simulink model "mcb_pmsm_foc_inductive_position_dsPIC33CK256MP508"  (R2023a)
settings: Solver=FixedStepDiscrete  StartTime=0.0  StopTime=10.0  FixedStep=50e-6  RelTol=1e-3  EnableMultiTasking=on
PreLoadFcn:
  | mcb_pmsm_foc_inductive_position_dsPIC33_data
PostLoadFcn:
  | mcb_pmsm_foc_inductive_position_dsPIC33_data
InitFcn:
  | mcb_pmsm_foc_inductive_position_dsPIC33_data
values from neighbouring files (symbols this model uses):
  PI_params = mcb.internal.SetControllerParameters(pmsm,inverter,PU_System,T_pwm,Ts,Ts_speed)    [dsPIC33CK256MP508_IPS_LVMC_sh.m]    (also in mcb_pmsm_foc_inductive_position_dsPIC33_data.m)
  PU_System = mcb_SetPUSystem(pmsm,inverter)    [dsPIC33CK256MP508_IPS_LVMC_sh.m]    (also in mcb_pmsm_foc_inductive_position_dsPIC33_data.m)
  PWM_frequency = 20e3    (= 20000)    [dsPIC33CK256MP508_IPS_LVMC_sh.m]    (also in mcb_pmsm_foc_inductive_position_dsPIC33_data.m)
  Ts = T_pwm    (= 5e-05)    [dsPIC33CK256MP508_IPS_LVMC_sh.m]    (also in mcb_pmsm_foc_inductive_position_dsPIC33_data.m)
  Ts_speed = 30*Ts    (= 0.0015)    [dsPIC33CK256MP508_IPS_LVMC_sh.m]    (also in mcb_pmsm_foc_inductive_position_dsPIC33_data.m)
undefined symbols (not defined in the file or in its folder): A0, A4, AN0, AN1, B0, B2, C12, C13, C14, C7, D11, D12, D13, D14, D5, D6, D7, DiscIntNeverNeededParam, inverter, Max, MaxPer, ms, NumBits1, NumBits2, P20, P32, P55, P60, P61, P62, P69, P70, P71, P75, P76, P77, P78, Pin, pmsm, PWM1max, Resol, s, us
libraries: simulink x29, MCHP_Blockset x22, mcbcontrolslib x7, slpidlib x3
(part 1 of 4)
settings Model: ExtModeBatchMode=on  ExtModeEnableFloating=off  ExtModeTrigDuration=32  Creator=I50990  LastModifiedBy=I50990
settings SolverCC: AutoInsertRateTranBlk=on
settings OptimizationCC: DefaultParameterBehavior=Inlined  DefaultUnderspecifiedDataType=single  InlineInvariantSignals=on  ReuseModelBlockBuffer=off  EnhancedBackFolding=on  StrengthReduction=on  BooleansAsBitfields=on  PassReuseOutputArgsAs=Individual arguments  ZeroExternalMemoryAtStartup=off  ZeroInternalMemoryAtStartup=off  OptimizeBlockOrder=speed  DifferentSizesBufferReuse=on  EfficientTunableParamExpr=on
settings DebuggingCC: MultiTaskDSMMsg=none  MultiTaskCondExecSysMsg=none  MultiTaskRateTransMsg=warning  ParameterOverflowMsg=none  ParameterPrecisionLossMsg=none  ParameterTunabilityLossMsg=error
settings HardwareCC: ProdBitPerInt=16  ProdBitPerPointer=16  ProdBitPerSizeT=16  ProdBitPerPtrDiffT=32  ProdLargestAtomicInteger=Integer  ProdLargestAtomicFloat=None  ProdWordSize=16  ProdLongLongMode=on  ProdHWDeviceType=Generic->Custom
settings ModelReferenceCC: ModelReferenceNumInstancesAllowed=Single
settings SFSimCC: MATLABDynamicMemAlloc=off
settings RTWCC: Description=Microchip Embedded Target PIC24 dsPIC30 dsPIC33 (real-time)  SystemTargetFile=MCHP_dsPIC_stf.tlc  TLCOptions="-aExtModeXCPClassicInterface=0  -aCreateExtModeTypes=1 -aExtModeXCPSimulationTimeInTicks=1"  TemplateMakefile=MCHP_dsPIC.tmf
settings CodeAppCC: ForceParamTrailComments=on  IgnoreCustomStorageClasses=off  MaxIdLength=255  OperatorAnnotations=on  SimulinkDataObjDesc=on  SFDataObjDesc=on  InsertBlockDesc=on
settings STFCustomTargetCC: TargetLibSuffix=_lib.a  TargetLangStandard=C89/C90 (ANSI)  CodeReplacementLibrary=Microchip Code Replacement Library for dsPIC  MultiwordLength=256  ConcurrentExecutionCompliant=off  CombineOutputUpdateFcns=on  CombineSignalStateStructs=on  SuppressErrorStatus=on  ERTCustomFileBanners=on  SupportNonFinite=off  SupportContinuousTime=off  RemoveResetFunc=on  MATLABClassNameForMDSCustomization=Simulink.SoftwareTarget.ERTCustomization  GRTInterface=off  UseToolchainInfoCompliant=off  SystemTargetFile=MCHP_dsPIC_stf.tlc
settings ERTTargetCC: TargetLibSuffix=_lib.a  CodeReplacementLibrary=Microchip Code Replacement Library for dsPIC  ParMdlRefBuildCompliant=off  CompOptLevelCompliant=off  ConcurrentExecutionCompliant=off  CombineSignalStateStructs=on  SuppressErrorStatus=on  SupportNonFinite=off  SupportNonInlinedSFcns=on  ModelStepFunctionPrototypeControlCompliant=off  CPPClassGenCompliant=off  UseToolchainInfoCompliant=off  ExtModeTransport=1  ExtModeStaticAlloc=on  ExtModeAutomaticAllocSize=off  ExtModeStaticAllocSize=2048  ExtModeMexFile=ext_xcp  ExtModeMexArgs=1 0 4000000 './MCHP_LVMC_template.X/MCHP_LVMC_template.elf'  ExtModeIntrfLevel=Level2 - Open  InlinedParameterPlacement=NonHierarchical  ERTSrcFileBannerTemplate=MCHP_dsPIC_code_template.cgt  ERTHdrFileBannerTemplate=MCHP_dsPIC_code_template.cgt  ERTDataSrcFileTemplate=MCHP_dsPIC_code_template.cgt  ERTDataHdrFileTemplate=MCHP_dsPIC_code_template.cgt  ERTCustomFileTemplate=MCHP_main.tlc  MaxLineWidth=110

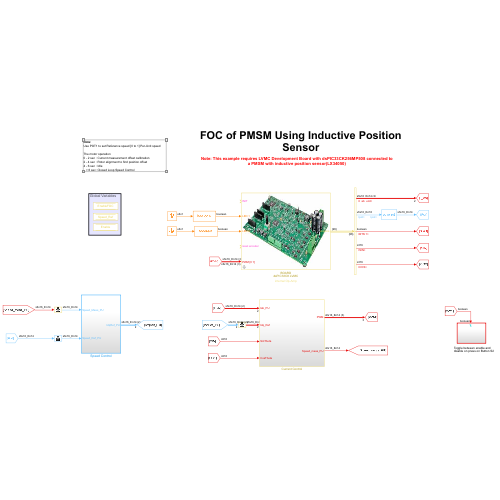
[thumbnail: Simulink's stored preview of the top-level diagram]
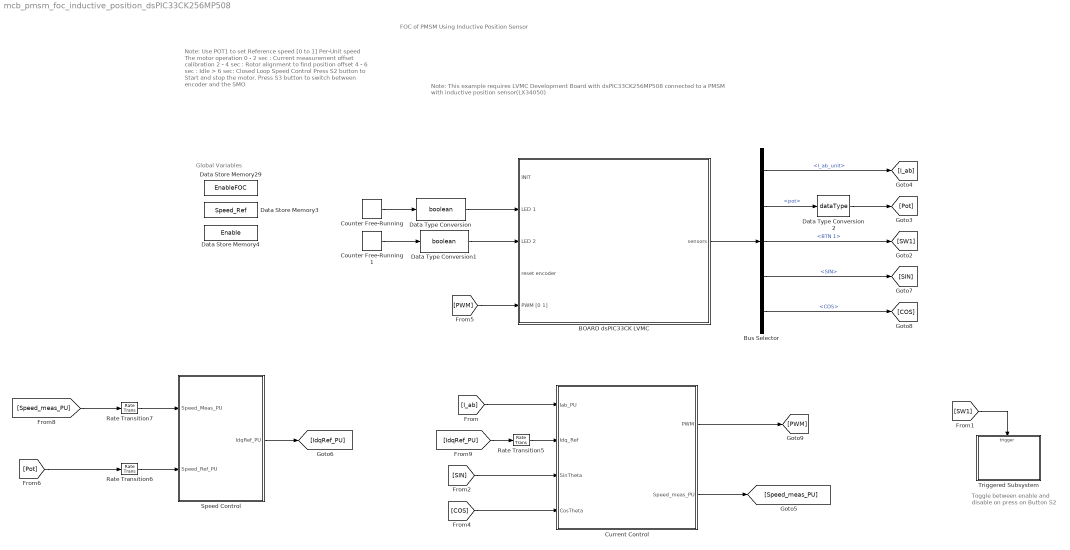
== system mcb_pmsm_foc_inductive_position_dsPIC33CK256MP508 ==
  note: Note:
      | Use POT1 to set Reference speed [0 to 1] Per-Unit speed
      |
      | The motor operation
      | 0 - 2 sec : Current measurement offset calibration
      | 2 - 4 sec : Rotor alignment to find position offset
      | 4 - 6 sec : Idle
      | > 6 sec: Closed Loop Speed Control
      |
      | Press S2 button to Start and stop the motor.
      | Press S3 button to switch between encoder and the SMO
  note: FOC of PMSM Using Inductive Position Sensor
  note: Note: This example requires LVMC Development Board with dsPIC33CK256MP508 connected to a PMSM with inductive position sensor(LX34050)
  note: Toggle between enable and disable on press on Button S2
  note: Global Variables
  BOARD dsPIC33CK LVMC : Subsystem  mask(dsPIC33CK Low Voltage Motor Control Board (LVMC) - dsPIC33CK256MP508){boardVariants=internal Op-Amp, n=4, QEIResolution=4000, QEI_Reset=on index signal, QEI_Offset_settings=0, QEIOffset=0}
      mask prompts: boardVariants "board variants"; n "Motor poles pairs"; QEIResolution "Optical encoder resolution per mechanical rotation (lines)"; QEI_Reset "Optical encoder reset"; QEI_Offset_settings "Optical encoder offset (mechanical in rad)"; QEIOffset "Optical encoder offset (mechanical in rad)"
      mask help:
      | Template for motor control algorithm. Open subsystem (ctrl-u) for further customisation.
      |
      | Block bus output provices:
      |   - Current phase ia & ib, DC bus and potentiometer position
      |   - Buttons (0 when pressed)
      |   - QEI position and velocity
      |   - MCU load and overload
      |
      | Block inputs:
      |   - INIT signal average the current phase ia and ib to be removed
      |   - LEDs
      |   - Reset encoder allows to align the motor while reseting the encoder
      |   - PWM normalized duty cycle value
      |
      | Model 50us base rate (20kHz) is synchronized with ADC conversion which is synchronized with the 50us PWM periods
      mask init:
      | BlksQEI = find_system(gcb,'FollowLinks','on','LookUnderMasks','all','ReferenceBlock','MCHP_Blockset/QEI/QEI');
      | QEI_Reset = get_param(gcb,'QEI_Reset');
      | if numel(BlksQEI) >= 1
      |     switch QEI_Reset
      |         case 'on index signal'
      |             set_param(BlksQEI{1},'PIMOD_mode','RESET position on each INDEX event');
      |         case 'on logical input (software)'        
      |             set_param(BlksQEI{1},'PIMOD_mode','position is cyclique between user defined boundaries'); 
      |         case 'custom setting'
      |             % do nothing 
      |     end
      | end % if
      | 
      | 
      |     BlksOpAmp = find_system(gcb,'FollowLinks','on','IncludeCommented','on','LookUnderMasks','all','ReferenceBlock','MCHP_Blockset/Analog IO/Op-Amp');
      |     if numel(BlksOpAmp) >= 1
      |         boardVariants = get_param(gcb,'boardVariants');
      |         switch boardVariants
      |             case 'internal Op-Amp'
      |                 set_param(BlksOpAmp{1},'Commented','off');
      |             case 'external Op-Amp'
      |                 set_param(BlksOpAmp{1},'Commented','on');
      |         end
      |     end % if
      settings: AttributesFormatString=%<boardVariants>
      mask TypeOptions boardVariants: internal Op-Amp | external Op-Amp
      mask TypeOptions n: 1 | 2 | 3 | 4 | 5 | 6 | 7 | 8 | 9 | 10 | 11 | 12 | 13 | 14 | 15 | 16
      mask TypeOptions QEI_Reset: on index signal | on logical input (software) | custom setting
      mask Callback QEI_Reset:
      | QEI_Reset = get_param(gcb,'QEI_Reset');
      | switch QEI_Reset
      |     case 'on index signal'
      |         QEIOffset = MCHP_Fun.Evalin('base','QEIOffset');
      |         set_param(gcb,'QEIOffset',num2str(QEIOffset));
      |         set_param(gcb,'MaskVisibilities',{'on';'on';'on';'on';'on';'off'});
      |     case 'on logical input (software)'
      |         set_param(gcb,'QEIOffset','0');
      |         set_param(gcb,'MaskVisibilities',{'on';'on';'on';'on';'off';'off'});
      |     case 'custom setting'
      |         set_param(gcb,'MaskVisibilities',{'on';'on';'on';'on';'on';'off'});
      |         % do nothing
      | end
      mask DialogControl boardVariants Tooltip: Default board use internal Op-Amp
      mask DialogControl n Tooltip: Number of pole pairs of the motor
      mask DialogControl QEIResolution Tooltip: encoder resolution per mechanical rotation
      mask DialogControl QEI_Reset Tooltip: enable encoder index signal if available. Otherwise align motor by applying a tension and set the rst input to 1
      mask DialogControl QEI_Offset_settings Tooltip: offset angle between encoder index and motor winding reference axis applied on theta_m and theta_e
      mask Display: image('$imagefile'); % Use "Edit Image" on toolstrip to change.
  Bus Selector : BusSelector  OutputSignals=ADC_unit.I_ab_unit,ADC.pot,BTN.BTN 1,SIN,COS
  Counter Free-Running : simulink/Sources/Counter Free-Running  NumBits=1  tsamp=0.5
  Counter Free-Running1 : simulink/Sources/Counter Free-Running  NumBits=1  tsamp=0.1
  Current Control : Subsystem  VariantControl=Optimized
  Data Store Memory29 : DataStoreMemory  DataStoreName=EnableFOC  ShowAdditionalParam=off  OutDataTypeStr=boolean
  Data Store Memory3 : DataStoreMemory  DataStoreName=Speed_Ref  ShowAdditionalParam=off
  Data Store Memory4 : DataStoreMemory  DataStoreName=Enable  ShowAdditionalParam=off  OutDataTypeStr=boolean
  Data Type Conversion : DataTypeConversion  OutDataTypeStr=boolean  SaturateOnIntegerOverflow=off  RndMeth=Floor
  Data Type Conversion1 : DataTypeConversion  OutDataTypeStr=boolean  SaturateOnIntegerOverflow=off  RndMeth=Floor
  Data Type Conversion2 : DataTypeConversion  OutDataTypeStr=dataType  RndMeth=Simplest  SaturateOnIntegerOverflow=off
  Rate Transition5 : RateTransition  Deterministic=off
  Rate Transition6 : RateTransition  Deterministic=off
  Rate Transition7 : RateTransition  Deterministic=off
  Speed Control : Subsystem  TreatAsAtomicUnit=on
  Triggered Subsystem : Subsystem  TreatAsAtomicUnit=on
  wires:
  Counter Free-Running1/1 -> Data Type Conversion1/1
  Data Type Conversion1/1 -> BOARD dsPIC33CK LVMC/3(LED 2)
  Counter Free-Running/1 -> Data Type Conversion/1
  Data Type Conversion/1 -> BOARD dsPIC33CK LVMC/2(LED 1)
  [SW1] -> Triggered Subsystem/Trigger
  BOARD dsPIC33CK LVMC/1(sensors) -> Bus Selector/1
  Bus Selector/3 -> [SW1]  "<BTN 1>"
  Bus Selector/1 -> [I_ab]  "<I_ab_unit>"
  Data Type Conversion2/1 -> [Pot]
  Bus Selector/2 -> Data Type Conversion2/1  "<pot>"
  [PWM] -> BOARD dsPIC33CK LVMC/5(PWM [0 1])
  Bus Selector/4 -> [SIN]  "<SIN>"
  Bus Selector/5 -> [COS]  "<COS>"
  Current Control/1(PWM) -> [PWM]
  [IdqRef_PU] -> Rate Transition5/1
  Speed Control/1(IdqRef_PU) -> [IdqRef_PU]
  Rate Transition5/1 -> Current Control/2(Idq_Ref)
  [Speed_meas_PU] -> Rate Transition7/1
  Rate Transition7/1 -> Speed Control/1(Speed_Meas_PU)
  [I_ab] -> Current Control/1(Iab_PU)
  [SIN] -> Current Control/3(SinTheta)
  [COS] -> Current Control/4(CosTheta)
  [Pot] -> Rate Transition6/1
  Rate Transition6/1 -> Speed Control/2(Speed_Ref_PU)
  Current Control/2(Speed_meas_PU) -> [Speed_meas_PU]
